simulink model "findClosestPointOnPath_th"  (R2020a)
settings: Solver=VariableStepAuto  StartTime=0.0  StopTime=0  RelTol=1e-3
values from neighbouring files (symbols this model uses):
  aBooth = 0.4363    [findClosestPointOnPath_ts.m]    (also in findTargetPointOnPath_sFunc.m = block.InputPort(3).Data)
  bBooth = 0.9999    [findClosestPointOnPath_ts.m]    (also in findTargetPointOnPath_sFunc.m = block.InputPort(4).Data)
  G_rCM = [75;0;100]    [findClosestPointOnPath_ts.m]
  L1 = 50    [findClosestPointOnPath_ts.m]    (also in findTargetPointOnPath_sFunc.m = block.InputPort(1).Data)
  meanElev = 30*pi/180    (= 0.523598775598)    [findClosestPointOnPath_ts.m]
  radius = 150    [findClosestPointOnPath_ts.m]    (also in findTargetPointOnPath_sFunc.m = block.InputPort(6).Data)
  s0 = 0.75*2*pi    (= 4.71238898038)    [findClosestPointOnPath_ts.m]    (also in findTargetPointOnPath_sFunc.m = block.InputPort(2).Data)
libraries: calc_path_coordinates x2, findClosestPointOnPath x1, findTargetPathParameter x1
settings Model: Creator=Ayaz  LastModifiedBy=Ayaz

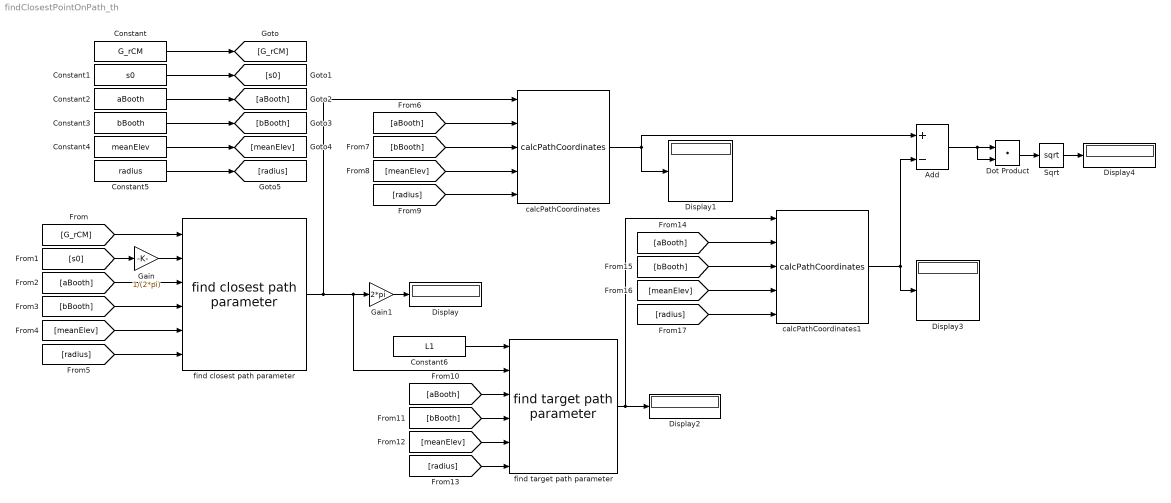
== system findClosestPointOnPath_th ==
  Add : Sum  Inputs=+-
  Constant : Constant  Value=G_rCM  VectorParams1D=off
  Constant1 : Constant  Value=s0  VectorParams1D=off
  Constant2 : Constant  Value=aBooth  VectorParams1D=off
  Constant3 : Constant  Value=bBooth  VectorParams1D=off
  Constant4 : Constant  Value=meanElev  VectorParams1D=off
  Constant5 : Constant  Value=radius  VectorParams1D=off
  Constant6 : Constant  Value=L1
  Display{,1..4} (5 alike) : Display
  Dot Product : DotProduct  InputSameDT=on  OutDataTypeStr=Inherit: Inherit via internal rule
  Gain : Gain  Gain=1/(2*pi)
  Gain1 : Gain  Gain=2*pi
  Sqrt : Sqrt  SaturateOnIntegerOverflow=on
  calcPathCoordinates : calc_path_coordinates/calcPathCoordinates  SystemSampleTime=-1  Latency=0  AutoFrameSizeCalculation=off
  calcPathCoordinates1 : calc_path_coordinates/calcPathCoordinates  SystemSampleTime=-1  Latency=0  AutoFrameSizeCalculation=off
  find closest path parameter : findClosestPointOnPath/find closest path parameter  maxBackward=0  maxForward=0.25  tau=0.618  convergeTol=convergeTol  MaxIters=25
  find target path parameter : findTargetPathParameter/find target path parameter  maxBackward=0  maxForward=0.25  tau=0.618  convergeTol=convergeTol  MaxIters=25
  wires:
  Constant/1 -> [G_rCM]
  Constant1/1 -> [s0]
  Constant2/1 -> [aBooth]
  Constant3/1 -> [bBooth]
  Constant4/1 -> [meanElev]
  Constant5/1 -> [radius]
  [G_rCM] -> find closest path parameter/1
  [radius] -> find closest path parameter/6
  [s0] -> Gain/1
  [aBooth] -> find closest path parameter/3
  [bBooth] -> find closest path parameter/4
  [meanElev] -> find closest path parameter/5
  [aBooth] -> calcPathCoordinates/2
  [bBooth] -> calcPathCoordinates/3
  [meanElev] -> calcPathCoordinates/4
  [radius] -> calcPathCoordinates/5
  find closest path parameter/1 -> calcPathCoordinates/1, find target path parameter/2, Gain1/1
  calcPathCoordinates/1 -> Display1/1, Add/1
  Constant6/1 -> find target path parameter/1
  [aBooth] -> find target path parameter/3
  [bBooth] -> find target path parameter/4
  [meanElev] -> find target path parameter/5
  [radius] -> find target path parameter/6
  find target path parameter/1 -> calcPathCoordinates1/1, Display2/1
  [radius] -> calcPathCoordinates1/5
  [meanElev] -> calcPathCoordinates1/4
  [bBooth] -> calcPathCoordinates1/3
  [aBooth] -> calcPathCoordinates1/2
  calcPathCoordinates1/1 -> Display3/1, Add/2
  Add/1 -> Dot Product/2, Dot Product/1
  Dot Product/1 -> Sqrt/1
  Sqrt/1 -> Display4/1
  Gain/1 -> find closest path parameter/2
  Gain1/1 -> Display/1
